simulink model "switching_table"  (R2015a)
settings: Solver=ode45  StartTime=0.0  StopTime=10.0  RelTol=1e-3
values from neighbouring files (symbols this model uses):
  sp00 = l.sp00    [power_control_param.m]    (also in sp00.mat = [1 1 1 1 1 0 0 0 0 0 0 1 ... (36 elements, 12x3)])
  sp01 = l.sp01    [power_control_param.m]    (also in sp01.mat = [1 1 1 0 0 0 0 0 0 1 1 1 ... (36 elements, 12x3)])
  sp10 = l.sp10    [power_control_param.m]    (also in sp10.mat = [1 1 1 0 1 1 0 0 0 1 0 0 ... (36 elements, 12x3)])
  sp11 = l.sp11    [power_control_param.m]    (also in sp11.mat = [1 1 0 0 1 1 0 0 1 1 0 0 ... (36 elements, 12x3)])
libraries: simulink x1
settings Model: Creator=rblan  LastModifiedBy=rblan

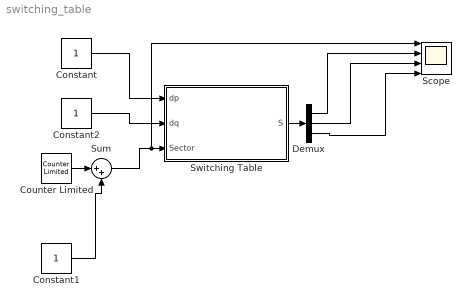
== system switching_table ==
  Constant : Constant
  Constant1 : Constant
  Constant2 : Constant
  Counter Limited : simulink/Sources/Counter Limited  uplimit=11  tsamp=-1
  Demux : Demux  Outputs=3
  Scope : Scope  NumInputPorts=4
      settings: YMin=0~0~0~0  YMax=12~1~1~1
  Sum : Sum  Inputs=|++
  "Switching Table " : Subsystem
  wires:
  "Switching Table "/1(S) -> Demux/1
  Demux/1 -> Scope/2
  Demux/2 -> Scope/3
  Demux/3 -> Scope/4
  Counter Limited/1 -> Sum/1
  Constant1/1 -> Sum/2
  Sum/1 -> Scope/1, "Switching Table "/3("Sector ")
  Constant/1 -> "Switching Table "/1(dp)
  Constant2/1 -> "Switching Table "/2(dq)

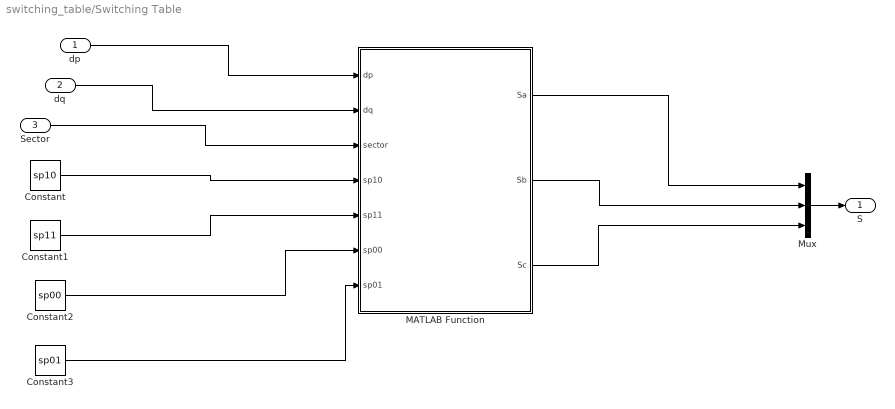
== system switching_table/Switching Table  ==
  dp : Inport
  dq : Inport  Port=2
  "Sector " : Inport  Port=3
  Constant : Constant  Value=sp10
  Constant1 : Constant  Value=sp11
  Constant2 : Constant  Value=sp00
  Constant3 : Constant  Value=sp01
  MATLAB Function : MATLAB Function  TreatAsAtomicUnit=on
  Mux : Mux  Inputs=3
  S : Outport
  wires:
  dp/1 -> MATLAB Function/1(dp)
  dq/1 -> MATLAB Function/2(dq)
  "Sector "/1 -> MATLAB Function/3(sector)
  MATLAB Function/2(Sb) -> Mux/2
  MATLAB Function/3(Sc) -> Mux/3
  Constant/1 -> MATLAB Function/4(sp10)
  Constant1/1 -> MATLAB Function/5(sp11)
  Constant2/1 -> MATLAB Function/6(sp00)
  Constant3/1 -> MATLAB Function/7(sp01)
  Mux/1 -> S/1
  MATLAB Function/1(Sa) -> Mux/1

== matlab function switching_table/Switching Table /MATLAB Function ==
  data: dp input; Sa output; dq input; sector input; Sb output; Sc output; sp10 input; sp11 input; sp00 input; sp01 input
function [Sa,Sb,Sc] = switch_selector(dp,dq,sector,sp10,sp11,sp00,sp01)
%#codegen
% global sp10 sp11 sp00 sp01
% 
% sp10= load('sp10.mat') ; 
% sp11=load('sp11.mat'); 
% sp00=load('sp00.mat');
% sp01 =load('sp01.mat'); 
%persistent Sa Sb Sc  
Sa= 0 ; 
Sb = 0 ; 
Sc = 0 ; 

switch dp
    case 1 
        switch dq
            case 0 
                Sa=sp10(sector,1) ; 
                Sb=sp10(sector,2) ; 
                Sc=sp10(sector,3) ; 
            case 1 
                Sa=sp11(sector,1) ; 
                Sb=sp11(sector,2) ; 
                Sc=sp11(sector,3) ; 
        end
    case 0 
        switch dq
            case 0 
                Sa=sp00(sector,1) ; 
                Sb=sp00(sector,2) ; 
                Sc=sp00(sector,3) ; 
            case 1 
                Sa=sp01(sector,1) ; 
                Sb=sp01(sector,2) ; 
                Sc=sp01(sector,3) ; 
        end
        
end
